simulink model "yek_be_liang"  (R2024a)
settings: Solver=VariableStepAuto  StartTime=0.0  StopTime=600  RelTol=1e-3
settings Model: Creator=MAHDI  LastModifiedBy=ASUS
settings SolverCC: AlgebraicLoopSolver=TrustRegion
settings DebuggingCC: UnconnectedInputMsg=warning  UnconnectedOutputMsg=warning  UnconnectedLineMsg=warning
settings ModelReferenceCC: EnableRefExpFcnMdlSchedulingChecks=on
settings RTWCC: GPUComputeCapability=3.5

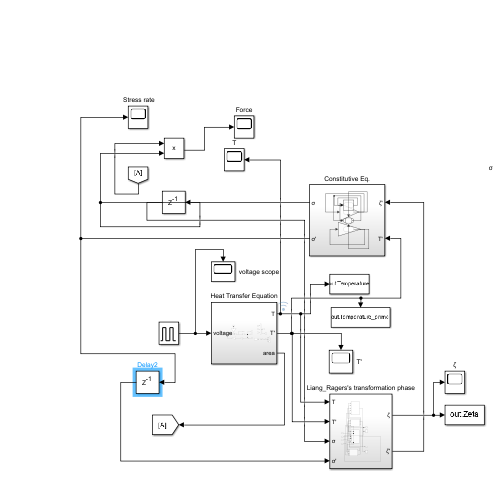
[thumbnail: Simulink's stored preview of the top-level diagram]
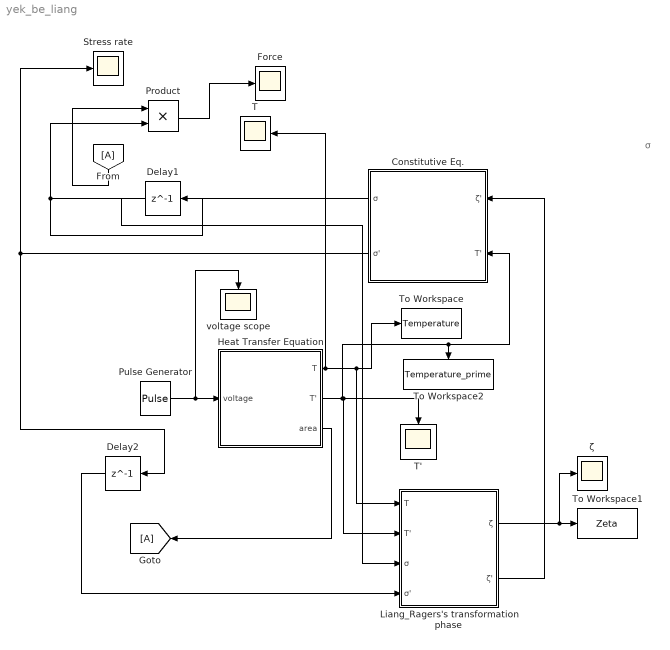
== system yek_be_liang ==
  note: σ
  " Stress rate" : Scope
  Constitutive Eq. : Subsystem
  Delay1 : Delay  DelayLength=1
  Delay2 : Delay  DelayLength=1
  Force : Scope
  From : From
  Goto : Goto
  Heat Transfer Equation : Subsystem
  Liang_Ragers's transformation phase : Subsystem
  Product : Product
  Pulse Generator : DiscretePulseGenerator  PulseType=Time based  Amplitude=50  Period=100  PulseWidth=50
  T : Scope
  T' : Scope
  To Workspace : ToWorkspace  VariableName=Temperature  SampleTime=1
  To Workspace1 : ToWorkspace  VariableName=Zeta  SampleTime=1
  To Workspace2 : ToWorkspace  VariableName=Temperature_prime  SampleTime=1
  voltage scope : Scope
  ζ : Scope
  wires:
  From/1 -> Product/1
  Delay1/1 -> Liang_Ragers's transformation phase/3(σ)
  Product/1 -> Force/1
  Constitutive Eq./2(σ') -> Delay2/1, " Stress rate"/1
  Pulse Generator/1 -> Heat Transfer Equation/1(voltage), voltage scope/1
  Delay2/1 -> Liang_Ragers's transformation phase/4("σ' ")
  Constitutive Eq./1(σ) -> Product/2, Delay1/1
  Heat Transfer Equation/1(T) -> Liang_Ragers's transformation phase/1(T), To Workspace/1, T/1
  Heat Transfer Equation/2(T') -> T'/1, Liang_Ragers's transformation phase/2(T'), Constitutive Eq./2(T'), To Workspace2/1
  Heat Transfer Equation/3(area) -> Goto/1
  Liang_Ragers's transformation phase/1(ζ) -> ζ/1, To Workspace1/1
  Liang_Ragers's transformation phase/2(ζ') -> Constitutive Eq./1(ζ')

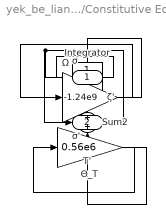
== system yek_be_liang/Constitutive Eq. ==
  ζ' : Inport
  T' : Inport  Port=2
  Integrator : Integrator
  Sum2 : Sum  Inputs=+|+
  Θ_T : Gain  Gain=0.56e6
  Ω : Gain  Gain=-1.24e9
  σ : Outport
  σ' : Outport  Port=2
  wires:
  T'/1 -> Θ_T/1
  ζ'/1 -> Ω/1
  Ω/1 -> Sum2/1
  Θ_T/1 -> Sum2/2
  Integrator/1 -> σ/1
  Sum2/1 -> Integrator/1, σ'/1

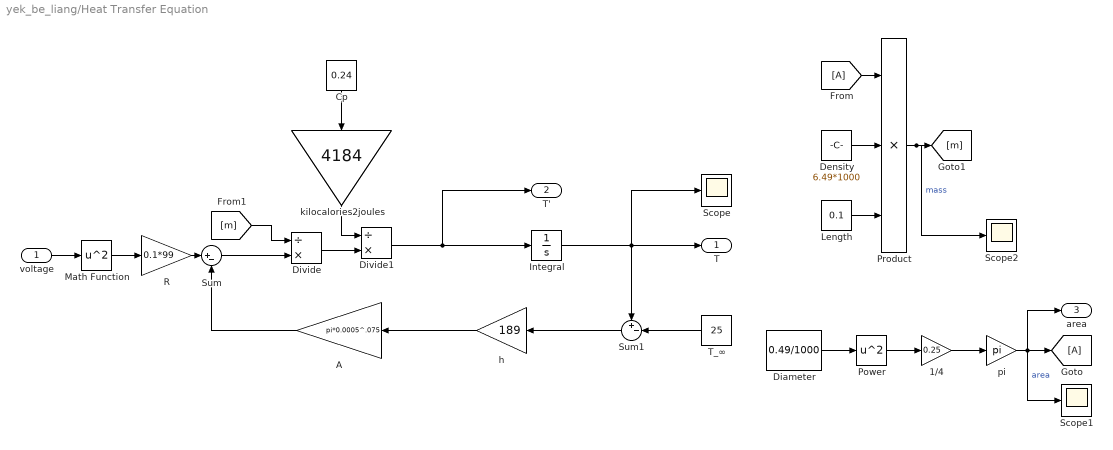
== system yek_be_liang/Heat Transfer Equation ==
  voltage : Inport
  1/4 : Gain  Gain=0.25
  A : Gain  Gain=pi*0.0005^.075
  Cp : Constant  Value=0.24
  Density : Constant  Value=6.49*1000
  Diameter : Constant  Value=0.49/1000
  Divide : Product  Inputs=/*
  Divide1 : Product  Inputs=/*
  From : From
  Goto : Goto
  Integral : Integrator  InitialCondition=25
  Length : Constant  Value=0.1
  Math Function : Math  Operator=square
  Power : Math  Operator=square
  Product : Product  Inputs=3
  R : Gain  Gain=0.1*99
  Scope : Scope
  Scope1 : Scope
  Scope2 : Scope
  Sum : Sum  Inputs=|+-
  Sum1 : Sum  Inputs=+-|
  T_∞ : Constant  Value=25
  h : Gain  Gain=189
  "kilocalories2joules " : Gain  Gain=4184
  pi : Gain  Gain=pi
  T : Outport
  T' : Outport  Port=2
  area : Outport  Port=3
  wires:
  T_∞/1 -> Sum1/2
  h/1 -> A/1
  Sum1/1 -> h/1
  Integral/1 -> Sum1/1, T/1, Scope/1
  R/1 -> Sum/1
  Math Function/1 -> R/1
  voltage/1 -> Math Function/1
  Product/1 -> Scope2/1, [m]  "mass"
  Sum/1 -> Divide/2
  Divide/1 -> Divide1/2
  Cp/1 -> "kilocalories2joules "/1
  "kilocalories2joules "/1 -> Divide1/1
  Divide1/1 -> T'/1, Integral/1
  Diameter/1 -> Power/1
  Power/1 -> 1/4/1
  1/4/1 -> pi/1
  Density/1 -> Product/2
  Length/1 -> Product/3
  pi/1 -> area/1, Scope1/1, Goto/1  "area"
  From/1 -> Product/1
  A/1 -> Sum/2
  [m] -> Divide/1

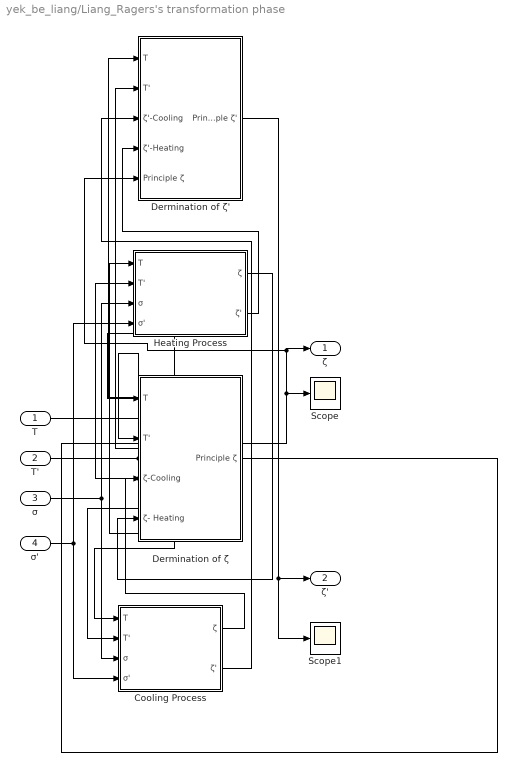
== system yek_be_liang/Liang_Ragers's transformation phase ==
  T : Inport
  T' : Inport  Port=2
  σ : Inport  Port=3
  "σ' " : Inport  Port=4
  Cooling Process : Subsystem
  Dermination of ζ : Subsystem
  Dermination of ζ' : Subsystem
  Heating Process : Subsystem
  Scope : Scope
  Scope1 : Scope
  ζ : Outport
  ζ' : Outport  Port=2
  wires:
  T/1 -> Dermination of ζ'/1(T), Dermination of ζ/1(T), Cooling Process/1(T), Heating Process/1(T)
  Dermination of ζ/1(Principle ζ) -> Dermination of ζ'/5(Principle ζ), ζ/1, Scope/1
  T'/1 -> Cooling Process/2(T'), Dermination of ζ'/2(T'), Heating Process/2(T'), Dermination of ζ/2(T')
  σ/1 -> Heating Process/3(σ), Cooling Process/3(σ)
  Cooling Process/2(ζ') -> Dermination of ζ'/3(ζ'-Cooling)
  Cooling Process/1(ζ) -> Dermination of ζ/3(ζ-Cooling)
  Heating Process/1(ζ) -> Dermination of ζ/4(ζ- Heating)
  Dermination of ζ'/1(Principle ζ') -> Scope1/1, ζ'/1
  Heating Process/2(ζ') -> Dermination of ζ'/4(ζ'-Heating)
  "σ' "/1 -> Heating Process/4("σ' "), Cooling Process/4("σ' ")

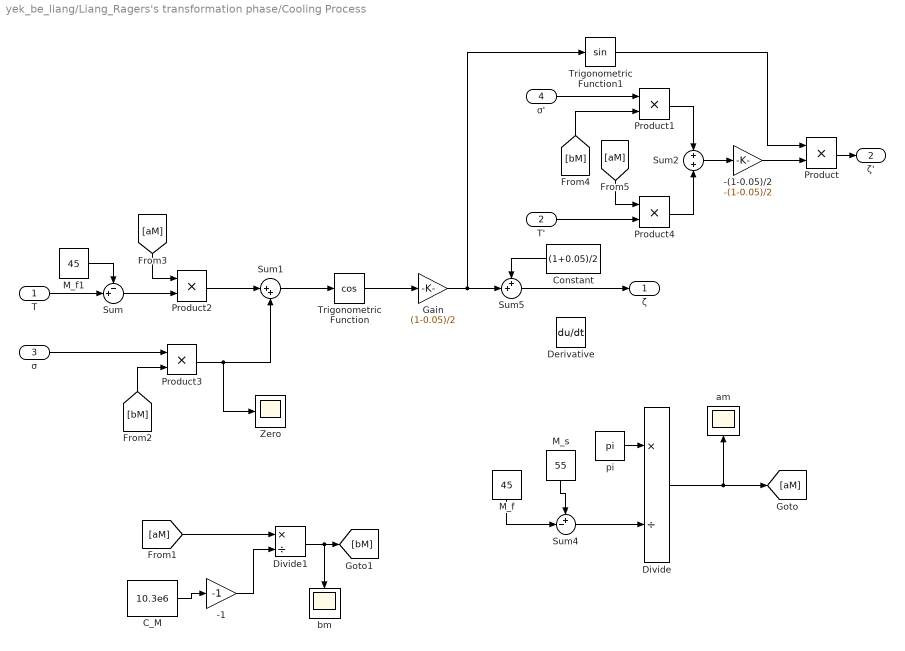
== system yek_be_liang/Liang_Ragers's transformation phase/Cooling Process ==
  T : Inport
  T' : Inport  Port=2
  σ : Inport  Port=3
  "σ' " : Inport  Port=4
  -(1-0.05)/2 : Gain  Gain=-(1-0.05)/2
  -1 : Gain  Gain=-1
  C_M : Constant  Value=10.3e6
  Constant : Constant  Value=(1+0.05)/2
  Derivative : Derivative
  Divide : Product  Inputs=*/
  Divide1 : Product  Inputs=*/
  Gain : Gain  Gain=(1-0.05)/2
  M_f : Constant  Value=45
  M_f1 : Constant  Value=45
  M_s : Constant  Value=55
  Product{,1..4} (5 alike) : Product
  Sum : Sum  Inputs=-+|
  Sum1 : Sum  Inputs=|++
  Sum2 : Sum  Inputs=+|+
  Sum4 : Sum  Inputs=+-|
  Sum5 : Sum  Inputs=++|
  Trigonometric Function : Trigonometry  Operator=cos
  Trigonometric Function1 : Trigonometry
  Zero : Scope
  am : Scope
  bm : Scope
  pi : Constant  Value=pi
  ζ : Outport
  ζ' : Outport  Port=2
  wires:
  Sum1/1 -> Trigonometric Function/1
  Trigonometric Function/1 -> Gain/1
  Sum5/1 -> ζ/1
  Constant/1 -> Sum5/1
  Gain/1 -> Trigonometric Function1/1, Sum5/2
  T/1 -> Sum/2
  Sum/1 -> Product2/2
  σ/1 -> Product3/1
  pi/1 -> Divide/1
  Sum4/1 -> Divide/2
  Divide/1 -> [aM], am/1
  C_M/1 -> -1/1
  [aM] -> Divide1/1
  -1/1 -> Divide1/2
  Divide1/1 -> [bM], bm/1
  [aM] -> Product2/1
  Product2/1 -> Sum1/1
  [bM] -> Product3/2
  Product3/1 -> Zero/1, Sum1/2
  [bM] -> Product1/2
  "σ' "/1 -> Product1/1
  [aM] -> Product4/1
  T'/1 -> Product4/2
  Product1/1 -> Sum2/1
  Product4/1 -> Sum2/2
  Product/1 -> ζ'/1
  M_s/1 -> Sum4/1
  M_f/1 -> Sum4/2
  Trigonometric Function1/1 -> Product/1
  Sum2/1 -> -(1-0.05)/2/1
  -(1-0.05)/2/1 -> Product/2
  M_f1/1 -> Sum/1

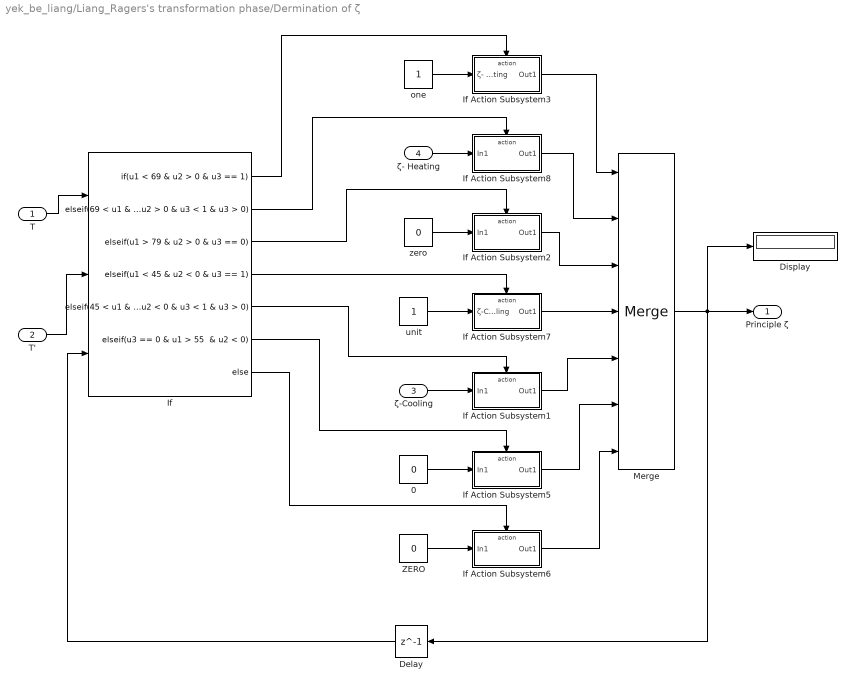
== system yek_be_liang/Liang_Ragers's transformation phase/Dermination of ζ ==
  T : Inport
  T' : Inport  Port=2
  ζ-Cooling : Inport  Port=3
  ζ- Heating : Inport  Port=4
  0 : Constant  Value=0
  Delay : Delay  DelayLength=1
  Display : Display
  If : If  NumInputs=3  IfExpression=u1 < 69 & u2 > 0 & u3 == 1  ElseIfExpressions="69 < u1 & u1 < 79  & u2 > 0 & u3 < 1 & u3 > 0 , u1 > 79 & u2 > 0 & u3 == 0, u1 < 45 & u2 < 0 & u3 == 1 , 45 < u1 & u1 < 55  & u2 < 0 & u3 < 1 & u3 > 0 , u3 == 0 & u1 > 55  & u2 < 0"
  If Action Subsystem1 : Subsystem  TreatAsAtomicUnit=on
  If Action Subsystem2 : Subsystem  TreatAsAtomicUnit=on
  If Action Subsystem3 : Subsystem  TreatAsAtomicUnit=on
  If Action Subsystem5 : Subsystem  TreatAsAtomicUnit=on
  If Action Subsystem6 : Subsystem  TreatAsAtomicUnit=on
  If Action Subsystem7 : Subsystem  TreatAsAtomicUnit=on
  If Action Subsystem8 : Subsystem  TreatAsAtomicUnit=on
  Merge : Merge  Inputs=7
  ZERO : Constant  Value=0
  one : Constant
  unit : Constant
  zero : Constant  Value=0
  Principle ζ : Outport
  wires:
  T/1 -> If/1
  T'/1 -> If/2
  If/1 -> If Action Subsystem3/Action
  If/2 -> If Action Subsystem8/Action
  If/3 -> If Action Subsystem2/Action
  If/4 -> If Action Subsystem7/Action
  If/5 -> If Action Subsystem1/Action
  If/6 -> If Action Subsystem5/Action
  If/7 -> If Action Subsystem6/Action
  ζ- Heating/1 -> If Action Subsystem8/1(In1)
  0/1 -> If Action Subsystem5/1(In1)
  ZERO/1 -> If Action Subsystem6/1(In1)
  zero/1 -> If Action Subsystem2/1(In1)
  If Action Subsystem7/1(Out1) -> Merge/4
  If Action Subsystem3/1(Out1) -> Merge/1
  If Action Subsystem8/1(Out1) -> Merge/2
  If Action Subsystem2/1(Out1) -> Merge/3
  If Action Subsystem1/1(Out1) -> Merge/5
  If Action Subsystem5/1(Out1) -> Merge/6
  If Action Subsystem6/1(Out1) -> Merge/7
  Merge/1 -> Delay/1, Display/1, Principle ζ/1
  ζ-Cooling/1 -> If Action Subsystem1/1(In1)
  one/1 -> If Action Subsystem3/1(ζ- Heating)
  unit/1 -> If Action Subsystem7/1(ζ-Cooling)
  Delay/1 -> If/3

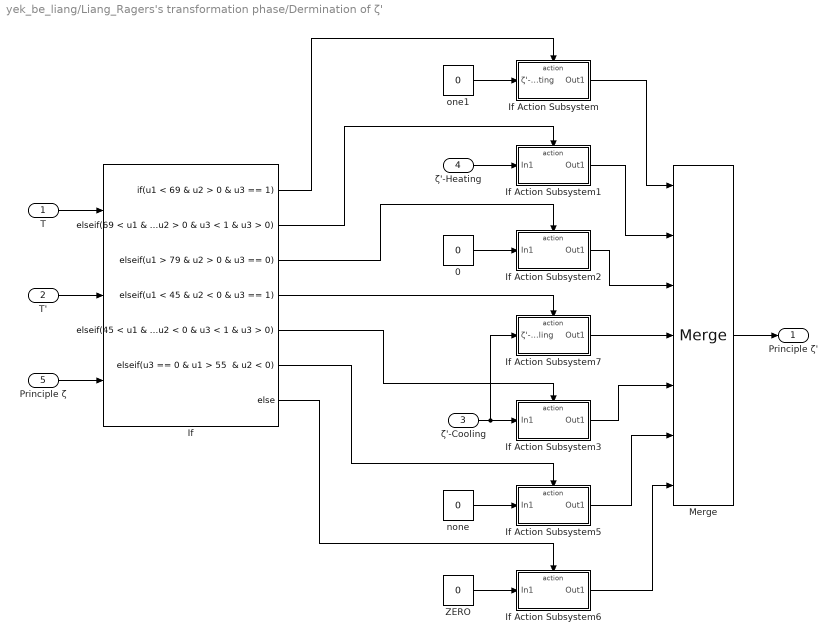
== system yek_be_liang/Liang_Ragers's transformation phase/Dermination of ζ' ==
  T : Inport
  T' : Inport  Port=2
  ζ'-Cooling : Inport  Port=3
  ζ'-Heating : Inport  Port=4
  Principle ζ : Inport  Port=5
  0 : Constant  Value=0
  If : If  NumInputs=3  IfExpression=u1 < 69 & u2 > 0 & u3 == 1  ElseIfExpressions="69 < u1 & u1 < 79  & u2 > 0 & u3 < 1 & u3 > 0 , u1 > 79 & u2 > 0 & u3 == 0, u1 < 45 & u2 < 0 & u3 == 1 , 45 < u1 & u1 < 55  & u2 < 0 & u3 < 1 & u3 > 0 , u3 == 0 & u1 > 55  & u2 < 0"
  If Action Subsystem : Subsystem  TreatAsAtomicUnit=on
  If Action Subsystem1 : Subsystem  TreatAsAtomicUnit=on
  If Action Subsystem2 : Subsystem  TreatAsAtomicUnit=on
  If Action Subsystem3 : Subsystem  TreatAsAtomicUnit=on
  If Action Subsystem5 : Subsystem  TreatAsAtomicUnit=on
  If Action Subsystem6 : Subsystem  TreatAsAtomicUnit=on
  If Action Subsystem7 : Subsystem  TreatAsAtomicUnit=on
  Merge : Merge  Inputs=7
  ZERO : Constant  Value=0
  none : Constant  Value=0
  one1 : Constant  Value=0
  Principle ζ' : Outport
  wires:
  Merge/1 -> Principle ζ'/1
  If Action Subsystem6/1(Out1) -> Merge/7
  If Action Subsystem5/1(Out1) -> Merge/6
  If Action Subsystem3/1(Out1) -> Merge/5
  If Action Subsystem2/1(Out1) -> Merge/3
  If Action Subsystem1/1(Out1) -> Merge/2
  If Action Subsystem/1(Out1) -> Merge/1
  If Action Subsystem7/1(Out1) -> Merge/4
  0/1 -> If Action Subsystem2/1(In1)
  ZERO/1 -> If Action Subsystem6/1(In1)
  none/1 -> If Action Subsystem5/1(In1)
  ζ'-Heating/1 -> If Action Subsystem1/1(In1)
  If/7 -> If Action Subsystem6/Action
  If/6 -> If Action Subsystem5/Action
  If/5 -> If Action Subsystem3/Action
  If/4 -> If Action Subsystem7/Action
  If/3 -> If Action Subsystem2/Action
  If/2 -> If Action Subsystem1/Action
  If/1 -> If Action Subsystem/Action
  T'/1 -> If/2
  T/1 -> If/1
  ζ'-Cooling/1 -> If Action Subsystem7/1(ζ'-Cooling), If Action Subsystem3/1(In1)
  one1/1 -> If Action Subsystem/1(ζ'-Heating)
  Principle ζ/1 -> If/3

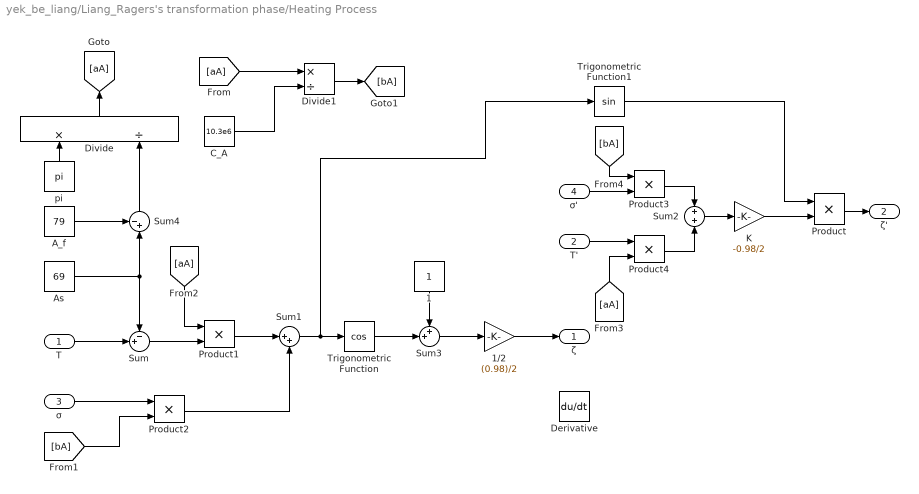
== system yek_be_liang/Liang_Ragers's transformation phase/Heating Process ==
  T : Inport
  T' : Inport  Port=2
  σ : Inport  Port=3
  "σ' " : Inport  Port=4
  1 : Constant
  1/2 : Gain  Gain=(0.98)/2
  A_f : Constant  Value=79
  As : Constant  Value=69
  C_A : Constant  Value=10.3e6
  Derivative : Derivative
  Divide : Product  Inputs=*/
  Divide1 : Product  Inputs=*/
  K : Gain  Gain=-0.98/2
  Product{,1..4} (5 alike) : Product
  Sum : Sum  Inputs=-+|
  Sum1 : Sum  Inputs=|++
  Sum2 : Sum  Inputs=+|+
  Sum3 : Sum  Inputs=++|
  Sum4 : Sum  Inputs=-+|
  Trigonometric Function : Trigonometry  Operator=cos
  Trigonometric Function1 : Trigonometry
  pi : Constant  Value=pi
  ζ : Outport
  ζ' : Outport  Port=2
  wires:
  As/1 -> Sum4/2, Sum/1
  T/1 -> Sum/2
  σ/1 -> Product2/1
  Sum1/1 -> Trigonometric Function1/1, Trigonometric Function/1
  Sum4/1 -> Divide/2
  pi/1 -> Divide/1
  Divide/1 -> [aA]
  A_f/1 -> Sum4/1
  [aA] -> Divide1/1
  C_A/1 -> Divide1/2
  Divide1/1 -> [bA]
  Sum/1 -> Product1/2
  [aA] -> Product1/1
  Product1/1 -> Sum1/1
  Product2/1 -> Sum1/2
  [bA] -> Product2/2
  "σ' "/1 -> Product3/2
  [bA] -> Product3/1
  T'/1 -> Product4/1
  [aA] -> Product4/2
  Product3/1 -> Sum2/1
  Product4/1 -> Sum2/2
  Product/1 -> ζ'/1
  Trigonometric Function/1 -> Sum3/2
  1/1 -> Sum3/1
  Sum3/1 -> 1/2/1
  1/2/1 -> ζ/1
  Trigonometric Function1/1 -> Product/1
  Sum2/1 -> K/1
  K/1 -> Product/2

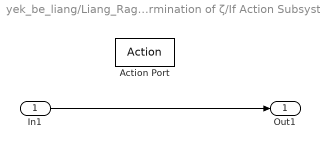
== system yek_be_liang/Liang_Ragers's transformation phase/Dermination of ζ/If Action Subsystem1 ==
  In1 : Inport
  Action Port : ActionPort  ActionPortLabel="elseif( 45 < u1 & u1 < 55  & u2 < 0 & u3 < 1 & u3 > 0 )"
  Out1 : Outport
  wires:
  In1/1 -> Out1/1

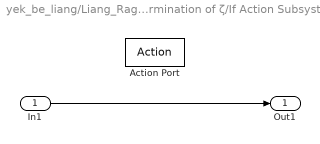
== system yek_be_liang/Liang_Ragers's transformation phase/Dermination of ζ/If Action Subsystem2 ==
  In1 : Inport
  Action Port : ActionPort  ActionPortLabel=elseif( u1 > 79 & u2 > 0 & u3 == 0)
  Out1 : Outport
  wires:
  In1/1 -> Out1/1

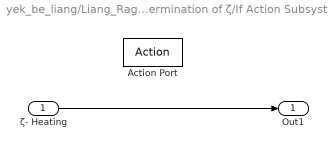
== system yek_be_liang/Liang_Ragers's transformation phase/Dermination of ζ/If Action Subsystem3 ==
  ζ- Heating : Inport
  Action Port : ActionPort  ActionPortLabel=if(u1 < 69 & u2 > 0 & u3 == 1)
  Out1 : Outport
  wires:
  ζ- Heating/1 -> Out1/1

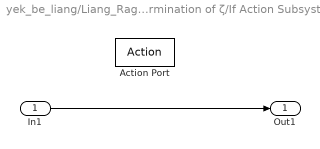
== system yek_be_liang/Liang_Ragers's transformation phase/Dermination of ζ/If Action Subsystem5 ==
  In1 : Inport
  Action Port : ActionPort  ActionPortLabel="elseif( u3 == 0 & u1 > 55  & u2 < 0)"
  Out1 : Outport
  wires:
  In1/1 -> Out1/1

== system yek_be_liang/Liang_Ragers's transformation phase/Dermination of ζ/If Action Subsystem6 ==
  In1 : Inport
  Action Port : ActionPort  ActionPortLabel=else
  Out1 : Outport
  wires:
  In1/1 -> Out1/1

== system yek_be_liang/Liang_Ragers's transformation phase/Dermination of ζ/If Action Subsystem7 ==
  ζ-Cooling : Inport
  Action Port : ActionPort  ActionPortLabel=elseif( u1 < 45 & u2 < 0 & u3 == 1 )
  Out1 : Outport
  wires:
  ζ-Cooling/1 -> Out1/1

== system yek_be_liang/Liang_Ragers's transformation phase/Dermination of ζ/If Action Subsystem8 ==
  In1 : Inport
  Action Port : ActionPort  ActionPortLabel="elseif(69 < u1 & u1 < 79  & u2 > 0 & u3 < 1 & u3 > 0 )"
  Out1 : Outport
  wires:
  In1/1 -> Out1/1

== system yek_be_liang/Liang_Ragers's transformation phase/Dermination of ζ'/If Action Subsystem ==
  ζ'-Heating : Inport
  Action Port : ActionPort  ActionPortLabel=if(u1 < 69 & u2 > 0 & u3 == 1)
  Out1 : Outport
  wires:
  ζ'-Heating/1 -> Out1/1

== system yek_be_liang/Liang_Ragers's transformation phase/Dermination of ζ'/If Action Subsystem1 ==
  In1 : Inport
  Action Port : ActionPort  ActionPortLabel="elseif(69 < u1 & u1 < 79  & u2 > 0 & u3 < 1 & u3 > 0 )"
  Out1 : Outport
  wires:
  In1/1 -> Out1/1

== system yek_be_liang/Liang_Ragers's transformation phase/Dermination of ζ'/If Action Subsystem2 ==
  In1 : Inport
  Action Port : ActionPort  ActionPortLabel=elseif( u1 > 79 & u2 > 0 & u3 == 0)
  Out1 : Outport
  wires:
  In1/1 -> Out1/1

== system yek_be_liang/Liang_Ragers's transformation phase/Dermination of ζ'/If Action Subsystem3 ==
  In1 : Inport
  Action Port : ActionPort  ActionPortLabel="elseif( 45 < u1 & u1 < 55  & u2 < 0 & u3 < 1 & u3 > 0 )"
  Out1 : Outport
  wires:
  In1/1 -> Out1/1

== system yek_be_liang/Liang_Ragers's transformation phase/Dermination of ζ'/If Action Subsystem5 ==
  In1 : Inport
  Action Port : ActionPort  ActionPortLabel="elseif( u3 == 0 & u1 > 55  & u2 < 0)"
  Out1 : Outport
  wires:
  In1/1 -> Out1/1

== system yek_be_liang/Liang_Ragers's transformation phase/Dermination of ζ'/If Action Subsystem6 ==
  In1 : Inport
  Action Port : ActionPort  ActionPortLabel=else
  Out1 : Outport
  wires:
  In1/1 -> Out1/1

== system yek_be_liang/Liang_Ragers's transformation phase/Dermination of ζ'/If Action Subsystem7 ==
  ζ'-Cooling : Inport
  Action Port : ActionPort  ActionPortLabel=elseif( u1 < 45 & u2 < 0 & u3 == 1 )
  Out1 : Outport
  wires:
  ζ'-Cooling/1 -> Out1/1
